simulink model "blockdemo"  (Simulink 6.3)
settings: Solver=FixedStepDiscrete  StartTime=0.0  StopTime=20  RelTol=1e-3
InitFcn:
  | %% DSPBuilder Start
  | alt_dspbuilder_update_model(bdroot)
  | %% DSPBuilder End
libraries: allblocks_alteradspbuilder2 x6
settings Model: Creator=mjervis  LastModifiedBy=delphick

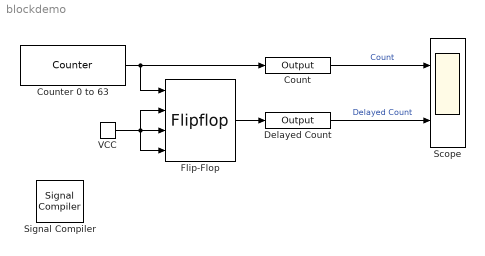
== system blockdemo ==
  Count : allblocks_alteradspbuilder2/Output  iofile=C:\workspace_clean\Documentation\DesignExamples\Tutorials\UnitBlocks\GateAndControl\FlipFlop\tb_blockdemo\blockdemo_Count.capture  BusType=Unsigned Integer  bwl=4  bwr=0  PORTTYPE=Output
  Counter 0 to 63 : allblocks_alteradspbuilder2/Counter  BusType=Unsigned Integer  bwl=4  bwr=0  use_modulo=on  modulo=64  SpecifyClock=off  direction=Increment  use_sload=off  use_sset=off  svalue=1  use_ena=off  use_sclr=off
  Delayed Count : allblocks_alteradspbuilder2/Output  iofile=C:\workspace_clean\Documentation\DesignExamples\Tutorials\UnitBlocks\GateAndControl\FlipFlop\tb_blockdemo\blockdemo_Delayed+Count.capture  BusType=Unsigned Integer  bwl=4  bwr=0  PORTTYPE=Output
  Flip-Flop : allblocks_alteradspbuilder2/Flipflop  mode=DFFE  BusType=Unsigned Integer  bwl=4  bwr=2
  Scope : Scope  NumInputPorts=2
      settings: TimeRange=20  YMin=0~0  YMax=16~16
  Signal Compiler : allblocks_alteradspbuilder2/Signal Compiler  DeviceFamily=Stratix IV  DeviceName=AUTO  EnableSignalTap=off  SignalTapDepth=128  UseBoardBlock=off  StpUseDefaultClock=on  StpClock=clock
  VCC : allblocks_alteradspbuilder2/VCC  SpecifyClock=off
  wires:
  Counter 0 to 63/1 -> Flip-Flop/1, Count/1
  Flip-Flop/1 -> Delayed Count/1
  Count/1 -> Scope/1  "Count"
  Delayed Count/1 -> Scope/2  "Delayed Count"
  VCC/1 -> Flip-Flop/4, Flip-Flop/3, Flip-Flop/2
